simulink model "ModeloNL"  (Simulink 7.7)
settings: Solver=ode45  StartTime=0.0  StopTime=10.0  RelTol=1e-3
values from neighbouring files (symbols this model uses):
  QT =     [FaseMinima.mat]    (also in FaseNaoMinima.mat; FaseNaoMinimaMudandoApenasGama.mat; settup.m = dynamics())
settings Model: Creator=Arthur  LastModifiedBy=Arthur

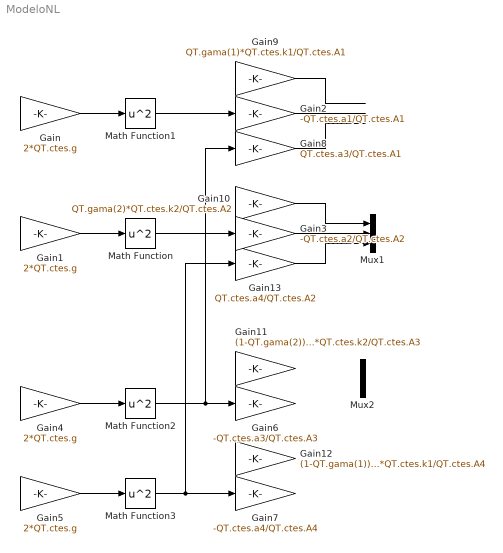
== system ModeloNL ==
  Gain{,1,4..5} (4 alike) : Gain  Gain=2*QT.ctes.g
  Gain10 : Gain  Gain=QT.gama(2)*QT.ctes.k2/QT.ctes.A2
  Gain11 : Gain  Gain=(1-QT.gama(2))*QT.ctes.k2/QT.ctes.A3
  Gain12 : Gain  Gain=(1-QT.gama(1))*QT.ctes.k1/QT.ctes.A4
  Gain13 : Gain  Gain=QT.ctes.a4/QT.ctes.A2
  Gain2 : Gain  Gain=-QT.ctes.a1/QT.ctes.A1
  Gain3 : Gain  Gain=-QT.ctes.a2/QT.ctes.A2
  Gain6 : Gain  Gain=-QT.ctes.a3/QT.ctes.A3
  Gain7 : Gain  Gain=-QT.ctes.a4/QT.ctes.A4
  Gain8 : Gain  Gain=QT.ctes.a3/QT.ctes.A1
  Gain9 : Gain  Gain=QT.gama(1)*QT.ctes.k1/QT.ctes.A1
  Math Function{,1..3} (4 alike) : Math  Operator=square  SaturateOnIntegerOverflow=on
  Mux1 : Mux  Inputs=3
  Mux2 : Mux  Inputs=2
  wires:
  Gain/1 -> Math Function1/1
  Gain1/1 -> Math Function/1
  Math Function1/1 -> Gain2/1
  Math Function/1 -> Gain3/1
  Gain4/1 -> Math Function2/1
  Math Function2/1 -> Gain6/1, Gain8/1
  Gain5/1 -> Math Function3/1
  Math Function3/1 -> Gain7/1, Gain13/1
  Gain9/1 -> ?
  Gain2/1 -> ?
  Gain8/1 -> ?
  Gain10/1 -> Mux1/1
  Gain3/1 -> Mux1/2
  Gain13/1 -> Mux1/3
